simulink model "BusWoObject"  (Simulink 7.4)
settings: Solver=ode45  StartTime=0.0  StopTime=10.0  RelTol=1e-3
settings Model: Creator=dread  LastModifiedBy=dread

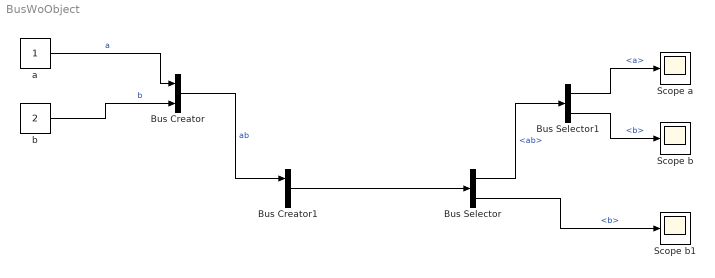
== system BusWoObject ==
  Bus Creator : BusCreator  Inputs=2
  Bus Creator1 : BusCreator  Inputs=2
  Bus Selector : BusSelector  OutputSignals=ab,ab.b
  Bus Selector1 : BusSelector  OutputSignals=a,b
  Scope a : Scope
  Scope b : Scope
  Scope b1 : Scope
      settings: SaveName=ScopeData2
  a : Constant  OutDataType=fixdt(1, 16)  OutScaling=2^0
  b : Constant  Value=2  OutDataType=fixdt(1, 16)  OutScaling=2^0
  wires:
  a/1 -> Bus Creator/1  "a"
  b/1 -> Bus Creator/2  "b"
  Bus Creator/1 -> Bus Creator1/1  "ab"
  Bus Selector/1 -> Bus Selector1/1  "<ab>"
  Bus Selector1/1 -> Scope a/1  "<a>"
  Bus Selector1/2 -> Scope b/1  "<b>"
  Bus Selector/2 -> Scope b1/1  "<b>"
  Bus Creator1/1 -> Bus Selector/1
